simulink model "AttitudePlayground"  (R2024b)
settings: Solver=FixedStepAuto  StartTime=0.0  StopTime=inf  FixedStep=delta_t  RelTol=1e-3  EnableMultiTasking=on
values from neighbouring files (symbols this model uses):
  A = [eye(3), delta_t * eye(3) ... (first row only)    [AttitudePlayground_Vars.m]    (also in ParameterIdentification.m = [0 1)
  A_ESO = [1-l1_ESO, delta_t-l1_ESO*delta_t ... (first row only)    [AttitudePlayground_Vars.m]
  A_kalman = [1 delta_t ... (first row only)    [AttitudePlayground_Vars.m]    (also in ControlSystem_Vars.m)
  acc_sigma = 0.2 * calc_sigma(acc_pp)    [AttitudePlayground_Vars.m]    (also in ControlSystem_Vars.m)
  alpha_comp_pitch = calc_alpha(0.1, delta_t)    [AttitudePlayground_Vars.m]
  alpha_comp_roll = calc_alpha(0.1, delta_t)    [AttitudePlayground_Vars.m]
  alpha_comp_yaw = calc_alpha(1, delta_t)    [AttitudePlayground_Vars.m]
  B = zeros(6,3)    [AttitudePlayground_Vars.m]    (also in ParameterIdentification.m = [0)
  b_ESO = [b0_ESO*delta_t - l1_ESO*b0_ESO*delta_t ... (first row only)    [AttitudePlayground_Vars.m]
  bias_0 = [0, 0, 0]    [AttitudePlayground_Vars.m]
  bias_sigma = 0.000000001    (= 1e-09)    [AttitudePlayground_Vars.m]
  C = eye(6)    [AttitudePlayground_Vars.m]    (also in ParameterIdentification.m = [1 0])
  C_kalman = eye(2)    [AttitudePlayground_Vars.m]    (also in ControlSystem_Vars.m)
  delta_t = 0.01    [AttitudePlayground_Vars.m]    (also in ControlSystem_Vars.m; ParameterIdentification.m = t2 - t1)
  gyro_sigma = 1*((pi/180) * (0.07))    (= 0.0012217304764)    [AttitudePlayground_Vars.m]    (also in ControlSystem_Vars.m)
  gyro_sigma_3d = [1*gyro_sigma, 1*gyro_sigma, gyro_sigma]    [AttitudePlayground_Vars.m]    (also in ControlSystem_Vars.m)
  k_i_mahony = 0.0057    [AttitudePlayground_Vars.m]
  k_p_mahony = 0.42    [AttitudePlayground_Vars.m]
  l = [l1_ESO, l2_ESO]'    [AttitudePlayground_Vars.m]
  mag_sigma = 0.8 * calc_sigma(mag_pp)    [AttitudePlayground_Vars.m]
  P_0 = eye(4)    [AttitudePlayground_Vars.m]    (also in ControlSystem_Vars.m)
  P_0_gb = eye(7)    [AttitudePlayground_Vars.m]
  q_init = [cos(initial_yaw/2), 0, 0, sin(initial_yaw/2)]    [AttitudePlayground_Vars.m]
  q_sigma = 0.001    [AttitudePlayground_Vars.m]    (also in ControlSystem_Vars.m)
  R = 1.8 * diag([0.001396263^2, 0.0016580628^2, 0.05^2, ((pi/180) *              (0.05))^2, ((pi/180) * (0.07))^2, ((pi/180) * (0.07))^2])    [AttitudePlayground_Vars.m]    (also in ControlSystem_Vars.m = 0.015625)
  R_kalman = diag([(calc_sigma(0.8))^2, (0.07)^2])    [AttitudePlayground_Vars.m]    (also in ControlSystem_Vars.m)
  r_qekf = 1/sqrt(cos(magnetic_dip_angle_theta)^2 +      sin(magnetic_dip_angle_theta)^2)  * transpose([cos(magnetic_dip_angle_theta),0, sin(magnetic_dip_angle_theta)])    [AttitudePlayground_Vars.m]
  step_time = 10    [AttitudePlayground_Vars.m]
  tau_pitch_comp = 0.5    [AttitudePlayground_Vars.m]
  tau_roll_comp = 0.5    [AttitudePlayground_Vars.m]
  tau_yaw_comp = 3    [AttitudePlayground_Vars.m]
  Ts = delta_t    (= 0.01)    [AttitudePlayground_Vars.m]
  Ts2 = delta_t/2    (= 0.005)    [AttitudePlayground_Vars.m]
  Ts_IMU = delta_t    (= 0.01)    [AttitudePlayground_Vars.m]
  voltage_divider_Vout_max = 1.728    [AttitudePlayground_Vars.m]
undefined symbols (not defined in the file or in its folder): DiscIntNeverNeededParam, Discrete, Newton, Raphson, Time
libraries: simulink_extras x26, dspsigops x5, bbblueActuatorLib x4, ctrlSharedLib x2, matrix_library x2, dspmathops x2, dspstat3 x1, bbblueSensorLib x1, simulink x1, dspfdesign x1, bbblueBasicLib x1, vrlib x1
(part 2 of 3)

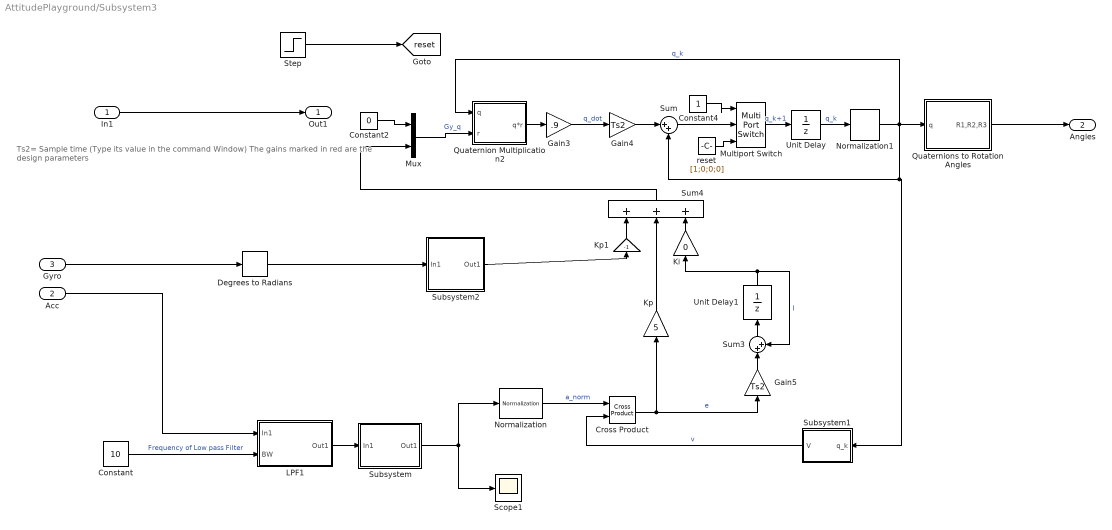
== system AttitudePlayground/Subsystem3 ==
  note: Ts2= Sample time (Type its value in the command Window)
      |
      | The gains marked in red are the design parameters
  In1 : Inport
  Acc : Inport  Port=2
  Gyro : Inport  Port=3
  Constant : Constant  Value=10
  Constant2 : Constant  Value=0
  Constant4 : Constant
  Cross Product : vrlib/Utilities/Cross Product
  Degrees to Radians : simulink_extras/Transformations/Degrees to Radians
  Gain3 : Gain  Gain=.9
  Gain4 : Gain  Gain=Ts2
  Gain5 : Gain  Gain=Ts2
  Ki : Gain  Gain=0
  Kp : Gain  Gain=5
  Kp1 : Gain  Gain=-1
  LPF1 : Subsystem
  Multiport Switch : MultiPortSwitch  Inputs=2  SaturateOnIntegerOverflow=off  InputSameDT=off
  Mux : Mux  Inputs=2
  Normalization : dspmathops/Normalization  NormType=Squared 2-norm  Bias=1e-10  NormOver=Each column  Dimension=1  roundingMode=Floor  overflowMode=off  accumDataTypeStr=Inherit: Same as product output  accumLastDataTypeStr=Inherit: Same as product output  outputDataTypeStr=Inherit: Same as product output  outputMin=[]  outputMax=[]  outputLastDataTypeStr=Inherit: Same as product output
  Normalization1 : dspmathops/Normalization  NormType=Squared 2-norm  Bias=1e-10  NormOver=Each column  Dimension=1  roundingMode=Floor  overflowMode=off  accumDataTypeStr=Inherit: Same as product output  accumLastDataTypeStr=Inherit: Same as product output  outputDataTypeStr=Inherit: Same as product output  outputMin=[]  outputMax=[]  outputLastDataTypeStr=Inherit: Same as product output
  Quaternion Multiplication2 : Subsystem
  Quaternions to Rotation Angles : Subsystem
  Scope1 : Scope
  Step : Step  Time=5  Before=2  SampleTime=delta_t
  Subsystem : Subsystem
  Subsystem1 : Subsystem
  Subsystem2 : Subsystem
  Sum : Sum  Inputs=|++
  Sum3 : Sum  Inputs=|++
  Sum4 : Sum  Inputs=+++
  Unit Delay : UnitDelay  InitialCondition=[1;0;0;0]  SampleTime=Ts  HasFrameUpgradeWarning=on
  Unit Delay1 : UnitDelay  InitialCondition=[0;0;0]  SampleTime=Ts  HasFrameUpgradeWarning=on
  reset : Constant  Value=[1;0;0;0]
  Out1 : Outport
  Angles : Outport  Port=2  VectorParamsAs1DForOutWhenUnconnected=off
  tag scope: reset=global
  wires:
  In1/1 -> Out1/1
  LPF1/1(Out1) -> Subsystem/1(In1)
  Sum4/1 -> Mux/2
  Gyro/1 -> Degrees to Radians/1
  Kp1/1 -> Sum4/1
  Ki/1 -> Sum4/3
  Unit Delay/1 -> Normalization1/1  "q_k"
  Subsystem2/1(Out1) -> Kp1/1
  reset/1 -> Multiport Switch/3
  Gain4/1 -> Sum/1
  Step/1 -> [reset]
  Unit Delay1/1 -> Ki/1, Sum3/2  "I"
  Constant4/1 -> Multiport Switch/1
  Sum/1 -> Multiport Switch/2
  Normalization/1 -> Cross Product/1  "a_norm"
  Constant/1 -> LPF1/2(BW)  "Frequency of Low pass Filter"
  Constant2/1 -> Mux/1
  Mux/1 -> Quaternion Multiplication2/2(r)  "Gy_q"
  Subsystem/1(Out1) -> Scope1/1, Normalization/1
  Gain3/1 -> Gain4/1  "q_dot"
  Quaternion Multiplication2/1(q*r) -> Gain3/1
  Degrees to Radians/1 -> Subsystem2/1(In1)
  Cross Product/1 -> Kp/1, Gain5/1  "e"
  Kp/1 -> Sum4/2
  Multiport Switch/1 -> Unit Delay/1  "q_k+1"
  Sum3/1 -> Unit Delay1/1
  Gain5/1 -> Sum3/1
  Subsystem1/1(V) -> Cross Product/2  "v"
  Acc/1 -> LPF1/1(In1)
  Quaternions to Rotation Angles/1(R1,R2,R3) -> Angles/1
  Normalization1/1 -> Quaternion Multiplication2/1(q), Quaternions to Rotation Angles/1(q), Subsystem1/1(q_k), Sum/2  "q_k"

== system AttitudePlayground/madgewick ==
  Gyroscope : Inport
  Out1 : Outport
  wires:
  Gyroscope/1 -> ?

== system AttitudePlayground/Angle_Accumulator_mat/Angle accumulator ==
  angle : Inport
  Bias : Bias  SaturateOnIntegerOverflow=off
  Constant4 : Constant
  Constant5 : Constant  Value=0
  Constant8 : Constant
  Constant9 : Constant  Value=0
  Gain : Gain  Gain=360
  Gain3 : Gain  Gain=-1
  Sum : Sum  Inputs=|++
  Sum1 : Sum  Inputs=|++
  Sum2 : Sum  Inputs=|-+
  Sum5 : Sum  Inputs=|++
  Sum6 : Sum  Inputs=+-|
  Switch : Switch  Criteria=u2 > Threshold  Threshold=180  SaturateOnIntegerOverflow=off  InputSameDT=off
  Switch1 : Switch  Criteria=u2 > Threshold  Threshold=180  SaturateOnIntegerOverflow=off  InputSameDT=off
  Unit Delay : UnitDelay  SampleTime=-1  HasFrameUpgradeWarning=on
  Unit Delay1 : UnitDelay  SampleTime=-1  HasFrameUpgradeWarning=on
  Unit Delay3 : UnitDelay  SampleTime=-1  HasFrameUpgradeWarning=on
  angle_acc : Outport
  wires:
  Sum1/1 -> Unit Delay/1, Sum6/1  "rot_amoun_fwt"
  Constant5/1 -> Switch/3
  Constant8/1 -> Switch1/1
  Sum5/1 -> Unit Delay3/1, Sum6/2
  Sum6/1 -> Gain/1
  Unit Delay/1 -> Sum1/2
  Constant4/1 -> Switch/1
  angle/1 -> Bias/1
  Unit Delay3/1 -> Sum5/2
  Switch/1 -> Sum1/1  "rot_done_fw"
  Sum2/1 -> Gain3/1, Switch/2
  Gain3/1 -> Switch1/2
  Unit Delay1/1 -> Sum2/2
  Sum/1 -> angle_acc/1  "abs_angle_deg"
  Switch1/1 -> Sum5/1  "rot_done_bw"
  Constant9/1 -> Switch1/3
  Gain/1 -> Sum/2
  Bias/1 -> Unit Delay1/1, Sum/1, Sum2/1

== system AttitudePlayground/Calculate RSME/Reset ==
  In1 : Inport  Partition=on  PartitionDimension=1  PartitionWidth=1  PartitionOffset=0
  For Each : ForEach  DisableCoverage=on
  Sample and Hold : dspsigops/Sample and Hold  trig=Rising edge  initCond=0  latchinput=off
  Step : Step  Time=step_time  SampleTime=0
  Sum : Sum  Inputs=|+-
  Out1 : Outport  ConcatenationDimension=1
  wires:
  In1/1 -> Sum/1, Sample and Hold/1
  Sample and Hold/1 -> Sum/2
  Step/1 -> Sample and Hold/Trigger
  Sum/1 -> Out1/1

== system AttitudePlayground/For Each Subsystem/Yaw accumulator ==
  yaw : Inport
  Bias : Bias  SaturateOnIntegerOverflow=off
  Constant4 : Constant
  Constant5 : Constant  Value=0
  Constant8 : Constant
  Constant9 : Constant  Value=0
  Gain : Gain  Gain=360
  Gain3 : Gain  Gain=-1
  Sum : Sum  Inputs=|++
  Sum1 : Sum  Inputs=|++
  Sum2 : Sum  Inputs=|-+
  Sum5 : Sum  Inputs=|++
  Sum6 : Sum  Inputs=+-|
  Switch : Switch  Criteria=u2 > Threshold  Threshold=180  SaturateOnIntegerOverflow=off  InputSameDT=off
  Switch1 : Switch  Criteria=u2 > Threshold  Threshold=180  SaturateOnIntegerOverflow=off  InputSameDT=off
  Unit Delay : UnitDelay  SampleTime=-1  HasFrameUpgradeWarning=on
  Unit Delay1 : UnitDelay  SampleTime=-1  HasFrameUpgradeWarning=on
  Unit Delay3 : UnitDelay  SampleTime=-1  HasFrameUpgradeWarning=on
  yaw_acc : Outport
  wires:
  Sum1/1 -> Unit Delay/1, Sum6/1  "rot_amoun_fwt"
  Constant5/1 -> Switch/3
  Constant8/1 -> Switch1/1
  Sum5/1 -> Unit Delay3/1, Sum6/2
  Sum6/1 -> Gain/1
  Unit Delay/1 -> Sum1/2
  Constant4/1 -> Switch/1
  yaw/1 -> Bias/1
  Unit Delay3/1 -> Sum5/2
  Switch/1 -> Sum1/1  "rot_done_fw"
  Sum2/1 -> Gain3/1, Switch/2
  Gain3/1 -> Switch1/2
  Unit Delay1/1 -> Sum2/2
  Sum/1 -> yaw_acc/1  "abs_angle_deg"
  Switch1/1 -> Sum5/1  "rot_done_bw"
  Constant9/1 -> Switch1/3
  Gain/1 -> Sum/2
  Bias/1 -> Unit Delay1/1, Sum/1, Sum2/1

== system AttitudePlayground/For Each Subsystem2/Yaw accumulator ==
  yaw : Inport
  Bias : Bias  SaturateOnIntegerOverflow=off
  Constant4 : Constant
  Constant5 : Constant  Value=0
  Constant8 : Constant
  Constant9 : Constant  Value=0
  Gain : Gain  Gain=360
  Gain3 : Gain  Gain=-1
  Sum : Sum  Inputs=|++
  Sum1 : Sum  Inputs=|++
  Sum2 : Sum  Inputs=|-+
  Sum5 : Sum  Inputs=|++
  Sum6 : Sum  Inputs=+-|
  Switch : Switch  Criteria=u2 > Threshold  Threshold=180  SaturateOnIntegerOverflow=off  InputSameDT=off
  Switch1 : Switch  Criteria=u2 > Threshold  Threshold=180  SaturateOnIntegerOverflow=off  InputSameDT=off
  Unit Delay : UnitDelay  SampleTime=-1  HasFrameUpgradeWarning=on
  Unit Delay1 : UnitDelay  SampleTime=-1  HasFrameUpgradeWarning=on
  Unit Delay3 : UnitDelay  SampleTime=-1  HasFrameUpgradeWarning=on
  yaw_acc : Outport
  wires:
  Sum1/1 -> Unit Delay/1, Sum6/1  "rot_amoun_fwt"
  Constant5/1 -> Switch/3
  Constant8/1 -> Switch1/1
  Sum5/1 -> Unit Delay3/1, Sum6/2
  Sum6/1 -> Gain/1
  Unit Delay/1 -> Sum1/2
  Constant4/1 -> Switch/1
  yaw/1 -> Bias/1
  Unit Delay3/1 -> Sum5/2
  Switch/1 -> Sum1/1  "rot_done_fw"
  Sum2/1 -> Gain3/1, Switch/2
  Gain3/1 -> Switch1/2
  Unit Delay1/1 -> Sum2/2
  Sum/1 -> yaw_acc/1  "abs_angle_deg"
  Switch1/1 -> Sum5/1  "rot_done_bw"
  Constant9/1 -> Switch1/3
  Gain/1 -> Sum/2
  Bias/1 -> Unit Delay1/1, Sum/1, Sum2/1

== system AttitudePlayground/Leightweight-Kalman/Yaw accumulator1 ==
  yaw : Inport
  Bias : Bias  SaturateOnIntegerOverflow=off
  Constant4 : Constant
  Constant5 : Constant  Value=0
  Constant8 : Constant
  Constant9 : Constant  Value=0
  Gain : Gain  Gain=360
  Gain3 : Gain  Gain=-1
  Sum : Sum  Inputs=|++
  Sum1 : Sum  Inputs=|++
  Sum2 : Sum  Inputs=|-+
  Sum5 : Sum  Inputs=|++
  Sum6 : Sum  Inputs=+-|
  Switch : Switch  Criteria=u2 > Threshold  Threshold=180  SaturateOnIntegerOverflow=off  InputSameDT=off
  Switch1 : Switch  Criteria=u2 > Threshold  Threshold=180  SaturateOnIntegerOverflow=off  InputSameDT=off
  Unit Delay : UnitDelay  SampleTime=-1  HasFrameUpgradeWarning=on
  Unit Delay1 : UnitDelay  SampleTime=-1  HasFrameUpgradeWarning=on
  Unit Delay3 : UnitDelay  SampleTime=-1  HasFrameUpgradeWarning=on
  yaw_acc : Outport
  wires:
  Sum1/1 -> Unit Delay/1, Sum6/1  "rot_amoun_fwt"
  Constant5/1 -> Switch/3
  Constant8/1 -> Switch1/1
  Sum5/1 -> Unit Delay3/1, Sum6/2
  Sum6/1 -> Gain/1
  Unit Delay/1 -> Sum1/2
  Constant4/1 -> Switch/1
  yaw/1 -> Bias/1
  Unit Delay3/1 -> Sum5/2
  Switch/1 -> Sum1/1  "rot_done_fw"
  Sum2/1 -> Gain3/1, Switch/2
  Gain3/1 -> Switch1/2
  Unit Delay1/1 -> Sum2/2
  Sum/1 -> yaw_acc/1  "abs_angle_deg"
  Switch1/1 -> Sum5/1  "rot_done_bw"
  Constant9/1 -> Switch1/3
  Gain/1 -> Sum/2
  Bias/1 -> Unit Delay1/1, Sum/1, Sum2/1

== system AttitudePlayground/Mahony Backup/Gyro - Bias - Removal ==
  In1 : Inport
  Constant1 : Constant  Value=0
  Constant3 : Constant
  Constant5 : Constant  Value=0
  Multiport Switch1 : MultiPortSwitch  Inputs=2  SaturateOnIntegerOverflow=off  InputSameDT=off
  Multiport Switch2 : MultiPortSwitch  Inputs=2  SaturateOnIntegerOverflow=off  InputSameDT=off
  Step : Step  Time=5  Before=2  SampleTime=Ts_IMU
  Subsystem3 : Subsystem
  Sum1 : Sum  Inputs=|+-
  Out1 : Outport  VectorParamsAs1DForOutWhenUnconnected=off
  tag scope: reset=global
  wires:
  [reset] -> Multiport Switch2/1
  In1/1 -> Subsystem3/1(Gyro), Sum1/1
  Constant3/1 -> Multiport Switch1/3
  Constant1/1 -> Multiport Switch1/2
  Sum1/1 -> Multiport Switch2/2
  Constant5/1 -> Multiport Switch2/3
  Multiport Switch1/1 -> Subsystem3/2(Switch)
  Subsystem3/1(Bias) -> Sum1/2
  [reset] -> Multiport Switch1/1
  Multiport Switch2/1 -> Out1/1
  Step/1 -> [reset]

== system AttitudePlayground/Mahony+Bias-Estimator/BIAS-ESO ==
  u : Inport
  Yaw_Fused : Inport  Port=2
  Gain : Gain  Gain=l
  Gain1 : Gain  Gain=b_ESO
  Gain2 : Gain  Gain=A_ESO  Multiplication=Matrix(K*u)
  Sum : Sum  Inputs=|++
  Sum1 : Sum  Inputs=++|
  Unit Delay : UnitDelay  SampleTime=delta_t  HasFrameUpgradeWarning=on
  Bias : Outport
  wires:
  Yaw_Fused/1 -> Gain/1
  u/1 -> Gain1/1
  Gain1/1 -> Sum/1
  Gain2/1 -> Sum/2
  Sum/1 -> Unit Delay/1
  Unit Delay/1 -> Sum1/1
  Gain/1 -> Sum1/2
  Sum1/1 -> Bias/1, Gain2/1  "x_hat"

== system AttitudePlayground/Mahony+Bias-Estimator/Gyro - Bias - Removal ==
  In1 : Inport
  Constant1 : Constant  Value=0
  Constant3 : Constant
  Constant5 : Constant  Value=0
  Multiport Switch1 : MultiPortSwitch  Inputs=2  SaturateOnIntegerOverflow=off  InputSameDT=off
  Multiport Switch2 : MultiPortSwitch  Inputs=2  SaturateOnIntegerOverflow=off  InputSameDT=off
  Step : Step  Time=step_time  Before=2  SampleTime=Ts_IMU
  Subsystem3 : Subsystem
  Sum1 : Sum  Inputs=|+-
  Out1 : Outport  VectorParamsAs1DForOutWhenUnconnected=off
  wires:
  Step/1 -> Multiport Switch2/1, Multiport Switch1/1
  In1/1 -> Subsystem3/1(Gyro), Sum1/1
  Constant3/1 -> Multiport Switch1/3
  Constant1/1 -> Multiport Switch1/2
  Sum1/1 -> Multiport Switch2/2
  Constant5/1 -> Multiport Switch2/3
  Multiport Switch1/1 -> Subsystem3/2(Switch)
  Subsystem3/1(Bias) -> Sum1/2
  Multiport Switch2/1 -> Out1/1

== system AttitudePlayground/Subsystem3/LPF1 ==
  In1 : Inport
  BW : Inport  Port=2
  Demux1 : Demux  Outputs=3
  LPF : Subsystem
  LPF1 : Subsystem
  LPF2 : Subsystem
  Mux1 : Mux  Inputs=3
  Out1 : Outport  VectorParamsAs1DForOutWhenUnconnected=off
  wires:
  In1/1 -> Demux1/1
  Demux1/2 -> LPF1/1(In)
  LPF1/1(Out1) -> Mux1/2
  BW/1 -> LPF2/2(BW), LPF1/2(BW), LPF/2(BW)
  LPF2/1(Out1) -> Mux1/3
  Demux1/3 -> LPF2/1(In)
  LPF/1(Out1) -> Mux1/1
  Mux1/1 -> Out1/1
  Demux1/1 -> LPF/1(In)

== system AttitudePlayground/Subsystem3/Quaternion Multiplication2 ==
  q : Inport  Unit=1
  r : Inport  Port=2  Unit=1
  Fcn : Fcn  Expr=u(5)*u(1) - u(6)*u(2) - u(7)*u(3) - u(8)*u(4)
  Fcn1 : Fcn  Expr=u(5)*u(2) + u(6)*u(1) - u(7)*u(4) + u(8)*u(3)
  Fcn2 : Fcn  Expr=u(5)*u(3) + u(6)*u(4) + u(7)*u(1) - u(8)*u(2)
  Fcn3 : Fcn  Expr=u(5)*u(4) - u(6)*u(3) + u(7)*u(2) + u(8)*u(1)
  Mux1 : Mux  Inputs=2
  Mux2 : Mux
  q*r : Outport  Unit=1  VectorParamsAs1DForOutWhenUnconnected=off
  wires:
  Mux1/1 -> Fcn3/1, Fcn2/1, Fcn/1, Fcn1/1
  Fcn/1 -> Mux2/1  "t0"
  Fcn1/1 -> Mux2/2  "t1"
  Fcn2/1 -> Mux2/3  "t2"
  Fcn3/1 -> Mux2/4  "t3"
  q/1 -> Mux1/1
  r/1 -> Mux1/2
  Mux2/1 -> q*r/1

== system AttitudePlayground/Subsystem3/Quaternions to Rotation Angles ==
  q : Inport  Unit=1
  Angle Calculation : Subsystem
  Quaternion Normalize : Subsystem
  fcn1 : Fcn  Expr=2*(u[2]*u[3] + u[1]*u[4])
  fcn2 : Fcn  Expr=u[1]*u[1] + u[2]*u[2] - u[3]*u[3] - u[4]*u[4]
  fcn3 : Fcn  Expr=-2*(u[2]*u[4] - u[1]*u[3])
  fcn4 : Fcn  Expr=2*(u[3]*u[4] + u[1]*u[2])
  fcn5 : Fcn  Expr=u[1]*u[1] - u[2]*u[2] - u[3]*u[3] + u[4]*u[4]
  R1,R2,R3 : Outport  Unit=rad  VectorParamsAs1DForOutWhenUnconnected=off
  wires:
  Quaternion Normalize/1(normal(q)) -> fcn3/1, fcn4/1, fcn5/1, fcn2/1, fcn1/1
  q/1 -> Angle Calculation/1(q), Quaternion Normalize/1(q)
  fcn2/1 -> Angle Calculation/3(r12)
  fcn3/1 -> Angle Calculation/4(r21)
  fcn5/1 -> Angle Calculation/6(r32)
  fcn4/1 -> Angle Calculation/5(In4)
  Angle Calculation/1(R1,R2,R3) -> R1,R2,R3/1
  fcn1/1 -> Angle Calculation/2(r11)

== system AttitudePlayground/Subsystem3/Subsystem ==
  In1 : Inport
  Constant6 : Constant  Value=0
  Constant7 : Constant
  Multiport Switch3 : MultiPortSwitch  Inputs=2  SaturateOnIntegerOverflow=off  InputSameDT=off
  Subsystem3 : Subsystem
  Sum2 : Sum  Inputs=|+-
  Out1 : Outport  VectorParamsAs1DForOutWhenUnconnected=off
  wires:
  Sum2/1 -> Out1/1
  Constant6/1 -> Multiport Switch3/2
  Subsystem3/1(Bias) -> Sum2/2
  In1/1 -> Sum2/1, Subsystem3/1(Accel)
  Multiport Switch3/1 -> Subsystem3/2(Switch)
  Constant7/1 -> Multiport Switch3/3
  [reset] -> Multiport Switch3/1

== system AttitudePlayground/Subsystem3/Subsystem1 ==
  q_k : Inport
  Fcn : Fcn  Expr=2*(u(2)*u(4)-u(1)*u(3))
  Fcn1 : Fcn  Expr=2*(u(1)*u(2)+u(3)*u(4))
  Fcn2 : Fcn  Expr=2*(0.5-u(2)^2-u(3)^2)
  Mux1 : Mux  Inputs=3
  V : Outport  VectorParamsAs1DForOutWhenUnconnected=off
  wires:
  Mux1/1 -> V/1
  Fcn2/1 -> Mux1/3
  Fcn1/1 -> Mux1/2
  q_k/1 -> Fcn2/1, Fcn1/1, Fcn/1
  Fcn/1 -> Mux1/1

== system AttitudePlayground/Subsystem3/Subsystem2 ==
  In1 : Inport
  Constant1 : Constant  Value=0
  Constant3 : Constant
  Constant5 : Constant  Value=0
  Multiport Switch1 : MultiPortSwitch  Inputs=2  SaturateOnIntegerOverflow=off  InputSameDT=off
  Multiport Switch2 : MultiPortSwitch  Inputs=2  SaturateOnIntegerOverflow=off  InputSameDT=off
  Subsystem3 : Subsystem
  Sum1 : Sum  Inputs=|+-
  Out1 : Outport  VectorParamsAs1DForOutWhenUnconnected=off
  wires:
  [reset] -> Multiport Switch2/1
  In1/1 -> Subsystem3/1(Gyro), Sum1/1
  Constant3/1 -> Multiport Switch1/3
  Constant1/1 -> Multiport Switch1/2
  Sum1/1 -> Multiport Switch2/2
  Constant5/1 -> Multiport Switch2/3
  Multiport Switch1/1 -> Subsystem3/2(Switch)
  Subsystem3/1(Bias) -> Sum1/2
  [reset] -> Multiport Switch1/1
  Multiport Switch2/1 -> Out1/1

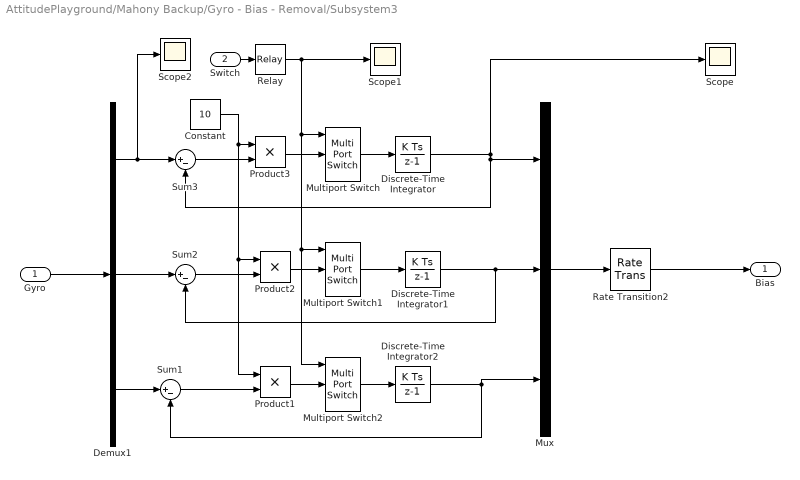
== system AttitudePlayground/Mahony Backup/Gyro - Bias - Removal/Subsystem3 ==
  Gyro : Inport
  Switch : Inport  Port=2
  Constant : Constant  Value=10
  Demux1 : Demux  Outputs=3
  Discrete-Time Integrator : DiscreteIntegrator  SampleTime=Ts_IMU  ICPrevOutput=DiscIntNeverNeededParam  ICPrevScaledInput=DiscIntNeverNeededParam
  Discrete-Time Integrator1 : DiscreteIntegrator  SampleTime=Ts_IMU  ICPrevOutput=DiscIntNeverNeededParam  ICPrevScaledInput=DiscIntNeverNeededParam
  Discrete-Time Integrator2 : DiscreteIntegrator  SampleTime=Ts_IMU  ICPrevOutput=DiscIntNeverNeededParam  ICPrevScaledInput=DiscIntNeverNeededParam
  Multiport Switch : MultiPortSwitch  Inputs=2  SaturateOnIntegerOverflow=off  InputSameDT=off
  Multiport Switch1 : MultiPortSwitch  Inputs=2  SaturateOnIntegerOverflow=off  InputSameDT=off
  Multiport Switch2 : MultiPortSwitch  Inputs=2  SaturateOnIntegerOverflow=off  InputSameDT=off
  Mux : Mux  Inputs=3
  Product1 : Product
  Product2 : Product
  Product3 : Product
  Rate Transition2 : RateTransition  OutPortSampleTime=Ts_IMU
  Relay : Relay  OnSwitchValue=.5  OffSwitchValue=.5  OffOutputValue=2
  Scope : Scope
  Scope1 : Scope
  Scope2 : Scope
  Sum1 : Sum  Inputs=|+-
  Sum2 : Sum  Inputs=|+-
  Sum3 : Sum  Inputs=|+-
  Bias : Outport  VectorParamsAs1DForOutWhenUnconnected=off
  wires:
  Gyro/1 -> Demux1/1
  Demux1/3 -> Sum1/1
  Product1/1 -> Multiport Switch2/2
  Sum1/1 -> Product1/2
  Multiport Switch2/1 -> Discrete-Time Integrator2/1
  Multiport Switch1/1 -> Discrete-Time Integrator1/1
  Sum2/1 -> Product2/2
  Product2/1 -> Multiport Switch1/2
  Demux1/2 -> Sum2/1
  Demux1/1 -> Scope2/1, Sum3/1
  Product3/1 -> Multiport Switch/2
  Sum3/1 -> Product3/2
  Discrete-Time Integrator/1 -> Sum3/2, Mux/1, Scope/1
  Constant/1 -> Product3/1, Product2/1, Product1/1
  Mux/1 -> Rate Transition2/1
  Multiport Switch/1 -> Discrete-Time Integrator/1
  Switch/1 -> Relay/1
  Relay/1 -> Scope1/1, Multiport Switch1/1, Multiport Switch2/1, Multiport Switch/1
  Rate Transition2/1 -> Bias/1
  Discrete-Time Integrator1/1 -> Sum2/2, Mux/2
  Discrete-Time Integrator2/1 -> Sum1/2, Mux/3

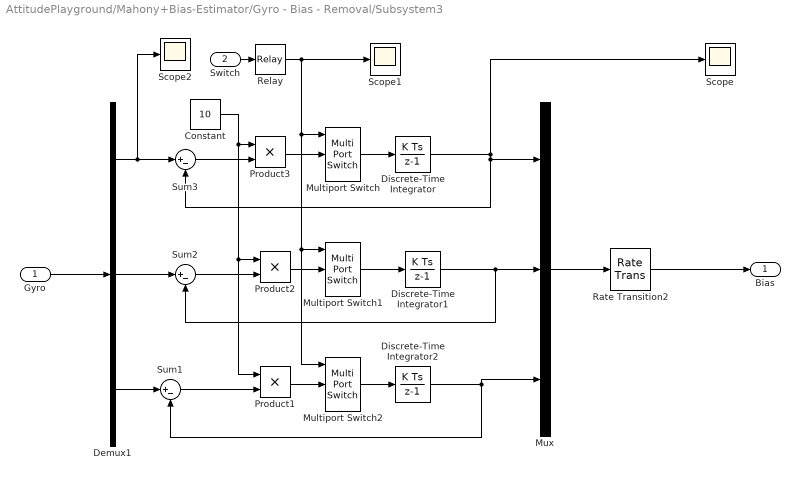
== system AttitudePlayground/Mahony+Bias-Estimator/Gyro - Bias - Removal/Subsystem3 ==
  Gyro : Inport
  Switch : Inport  Port=2
  Constant : Constant  Value=10
  Demux1 : Demux  Outputs=3
  Discrete-Time Integrator : DiscreteIntegrator  SampleTime=Ts_IMU  ICPrevOutput=DiscIntNeverNeededParam  ICPrevScaledInput=DiscIntNeverNeededParam
  Discrete-Time Integrator1 : DiscreteIntegrator  SampleTime=Ts_IMU  ICPrevOutput=DiscIntNeverNeededParam  ICPrevScaledInput=DiscIntNeverNeededParam
  Discrete-Time Integrator2 : DiscreteIntegrator  SampleTime=Ts_IMU  ICPrevOutput=DiscIntNeverNeededParam  ICPrevScaledInput=DiscIntNeverNeededParam
  Multiport Switch : MultiPortSwitch  Inputs=2  SaturateOnIntegerOverflow=off  InputSameDT=off
  Multiport Switch1 : MultiPortSwitch  Inputs=2  SaturateOnIntegerOverflow=off  InputSameDT=off
  Multiport Switch2 : MultiPortSwitch  Inputs=2  SaturateOnIntegerOverflow=off  InputSameDT=off
  Mux : Mux  Inputs=3
  Product1 : Product
  Product2 : Product
  Product3 : Product
  Rate Transition2 : RateTransition  OutPortSampleTime=Ts_IMU
  Relay : Relay  OnSwitchValue=.5  OffSwitchValue=.5  OffOutputValue=2
  Scope : Scope
  Scope1 : Scope
  Scope2 : Scope
  Sum1 : Sum  Inputs=|+-
  Sum2 : Sum  Inputs=|+-
  Sum3 : Sum  Inputs=|+-
  Bias : Outport  VectorParamsAs1DForOutWhenUnconnected=off
  wires:
  Gyro/1 -> Demux1/1
  Demux1/3 -> Sum1/1
  Product1/1 -> Multiport Switch2/2
  Sum1/1 -> Product1/2
  Multiport Switch2/1 -> Discrete-Time Integrator2/1
  Multiport Switch1/1 -> Discrete-Time Integrator1/1
  Sum2/1 -> Product2/2
  Product2/1 -> Multiport Switch1/2
  Demux1/2 -> Sum2/1
  Demux1/1 -> Scope2/1, Sum3/1
  Product3/1 -> Multiport Switch/2
  Sum3/1 -> Product3/2
  Discrete-Time Integrator/1 -> Sum3/2, Mux/1, Scope/1
  Constant/1 -> Product3/1, Product2/1, Product1/1
  Mux/1 -> Rate Transition2/1
  Multiport Switch/1 -> Discrete-Time Integrator/1
  Switch/1 -> Relay/1
  Relay/1 -> Scope1/1, Multiport Switch1/1, Multiport Switch2/1, Multiport Switch/1
  Rate Transition2/1 -> Bias/1
  Discrete-Time Integrator1/1 -> Sum2/2, Mux/2
  Discrete-Time Integrator2/1 -> Sum1/2, Mux/3

== system AttitudePlayground/Subsystem3/LPF1/LPF ==
  In : Inport
  BW : Inport  Port=2
  Discrete-Time Integrator : DiscreteIntegrator  SampleTime=Ts  ICPrevOutput=DiscIntNeverNeededParam  ICPrevScaledInput=DiscIntNeverNeededParam
  Product : Product
  Sum2 : Sum  Inputs=|+-
  Out1 : Outport  VectorParamsAs1DForOutWhenUnconnected=off
  wires:
  In/1 -> Sum2/1
  Sum2/1 -> Product/2
  Discrete-Time Integrator/1 -> Out1/1, Sum2/2
  Product/1 -> Discrete-Time Integrator/1
  BW/1 -> Product/1

== system AttitudePlayground/Subsystem3/LPF1/LPF1 ==
  In : Inport
  BW : Inport  Port=2
  Discrete-Time Integrator : DiscreteIntegrator  SampleTime=Ts  ICPrevOutput=DiscIntNeverNeededParam  ICPrevScaledInput=DiscIntNeverNeededParam
  Product : Product
  Sum2 : Sum  Inputs=|+-
  Out1 : Outport  VectorParamsAs1DForOutWhenUnconnected=off
  wires:
  BW/1 -> Product/1
  Product/1 -> Discrete-Time Integrator/1
  Discrete-Time Integrator/1 -> Sum2/2, Out1/1
  Sum2/1 -> Product/2
  In/1 -> Sum2/1

== system AttitudePlayground/Subsystem3/LPF1/LPF2 ==
  In : Inport
  BW : Inport  Port=2
  Discrete-Time Integrator : DiscreteIntegrator  SampleTime=Ts  ICPrevOutput=DiscIntNeverNeededParam  ICPrevScaledInput=DiscIntNeverNeededParam
  Product : Product
  Sum2 : Sum  Inputs=|+-
  Out1 : Outport  VectorParamsAs1DForOutWhenUnconnected=off
  wires:
  In/1 -> Sum2/1
  Sum2/1 -> Product/2
  Discrete-Time Integrator/1 -> Out1/1, Sum2/2
  Product/1 -> Discrete-Time Integrator/1
  BW/1 -> Product/1

== system AttitudePlayground/Subsystem3/Quaternions to Rotation Angles/Angle Calculation ==
  q : Inport
  r11 : Inport  Port=2
  r12 : Inport  Port=3
  r21 : Inport  Port=4
  In4 : Inport  Port=5
  r32 : Inport  Port=6
  Terminator : Terminator
  Trigonometric Function1 : Trigonometry  Operator=atan2
  Trigonometric Function3 : Trigonometry  Operator=atan2
  Vector Concatenate : Concatenate  NumInputs=3
  trigFcn : Trigonometry  Operator=asin
  R1,R2,R3 : Outport  VectorParamsAs1DForOutWhenUnconnected=off
  wires:
  Vector Concatenate/1 -> R1,R2,R3/1
  r11/1 -> Trigonometric Function1/1
  In4/1 -> Trigonometric Function3/1
  trigFcn/1 -> Vector Concatenate/2  "r2"
  r32/1 -> Trigonometric Function3/2
  r21/1 -> trigFcn/1
  Trigonometric Function3/1 -> Vector Concatenate/3  "r3"
  q/1 -> Terminator/1
  Trigonometric Function1/1 -> Vector Concatenate/1  "r1"
  r12/1 -> Trigonometric Function1/2

== system AttitudePlayground/Subsystem3/Quaternions to Rotation Angles/Quaternion Normalize ==
  q : Inport  Unit=1
  Demux : Demux
  Mux : Mux
  Product{,1..3} (4 alike) : Product  Inputs=*/
  Quaternion Modulus : Subsystem
  normal(q) : Outport  Unit=1  VectorParamsAs1DForOutWhenUnconnected=off
  wires:
  Product/1 -> Mux/1
  Product1/1 -> Mux/2
  Demux/1 -> Product/1
  Demux/2 -> Product1/1
  q/1 -> Quaternion Modulus/1(q), Demux/1
  Demux/4 -> Product3/1
  Mux/1 -> normal(q)/1
  Demux/3 -> Product2/1
  Product3/1 -> Mux/4
  Product2/1 -> Mux/3
  Quaternion Modulus/1(|q|) -> Product3/2, Product2/2, Product/2, Product1/2

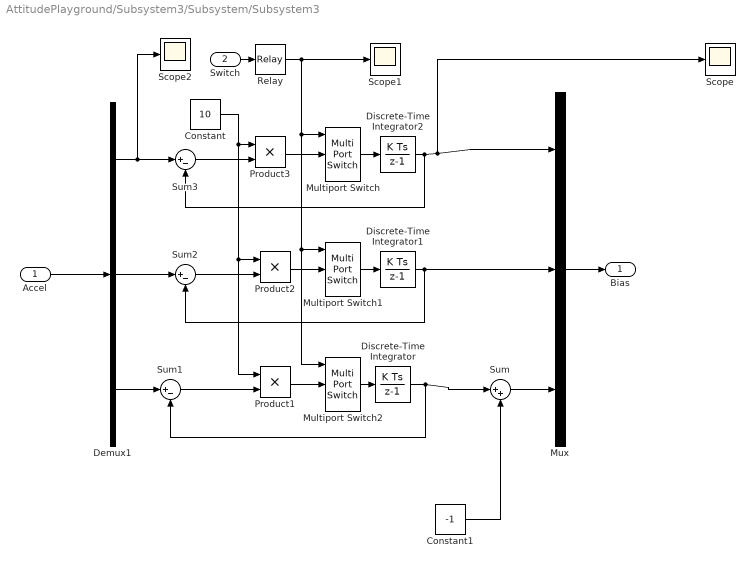
== system AttitudePlayground/Subsystem3/Subsystem/Subsystem3 ==
  Accel : Inport
  Switch : Inport  Port=2
  Constant : Constant  Value=10
  Constant1 : Constant  Value=-1
  Demux1 : Demux  Outputs=3
  Discrete-Time Integrator : DiscreteIntegrator  SampleTime=delta_t  ICPrevOutput=DiscIntNeverNeededParam  ICPrevScaledInput=DiscIntNeverNeededParam
  Discrete-Time Integrator1 : DiscreteIntegrator  SampleTime=delta_t  ICPrevOutput=DiscIntNeverNeededParam  ICPrevScaledInput=DiscIntNeverNeededParam
  Discrete-Time Integrator2 : DiscreteIntegrator  SampleTime=delta_t  ICPrevOutput=DiscIntNeverNeededParam  ICPrevScaledInput=DiscIntNeverNeededParam
  Multiport Switch : MultiPortSwitch  Inputs=2  SaturateOnIntegerOverflow=off  InputSameDT=off
  Multiport Switch1 : MultiPortSwitch  Inputs=2  SaturateOnIntegerOverflow=off  InputSameDT=off
  Multiport Switch2 : MultiPortSwitch  Inputs=2  SaturateOnIntegerOverflow=off  InputSameDT=off
  Mux : Mux  Inputs=3
  Product1 : Product
  Product2 : Product
  Product3 : Product
  Relay : Relay  OnSwitchValue=.5  OffSwitchValue=.5  OffOutputValue=2
  Scope : Scope
  Scope1 : Scope
  Scope2 : Scope
  Sum : Sum  Inputs=|++
  Sum1 : Sum  Inputs=|+-
  Sum2 : Sum  Inputs=|+-
  Sum3 : Sum  Inputs=|+-
  Bias : Outport  VectorParamsAs1DForOutWhenUnconnected=off
  wires:
  Accel/1 -> Demux1/1
  Demux1/3 -> Sum1/1
  Product1/1 -> Multiport Switch2/2
  Sum1/1 -> Product1/2
  Discrete-Time Integrator/1 -> Sum/1, Sum1/2
  Discrete-Time Integrator1/1 -> Mux/2, Sum2/2
  Sum2/1 -> Product2/2
  Product2/1 -> Multiport Switch1/2
  Demux1/2 -> Sum2/1
  Demux1/1 -> Scope2/1, Sum3/1
  Product3/1 -> Multiport Switch/2
  Sum3/1 -> Product3/2
  Discrete-Time Integrator2/1 -> Scope/1, Mux/1, Sum3/2
  Constant/1 -> Product3/1, Product2/1, Product1/1
  Mux/1 -> Bias/1
  Multiport Switch/1 -> Discrete-Time Integrator2/1
  Multiport Switch1/1 -> Discrete-Time Integrator1/1
  Multiport Switch2/1 -> Discrete-Time Integrator/1
  Switch/1 -> Relay/1
  Relay/1 -> Scope1/1, Multiport Switch1/1, Multiport Switch2/1, Multiport Switch/1
  Sum/1 -> Mux/3
  Constant1/1 -> Sum/2

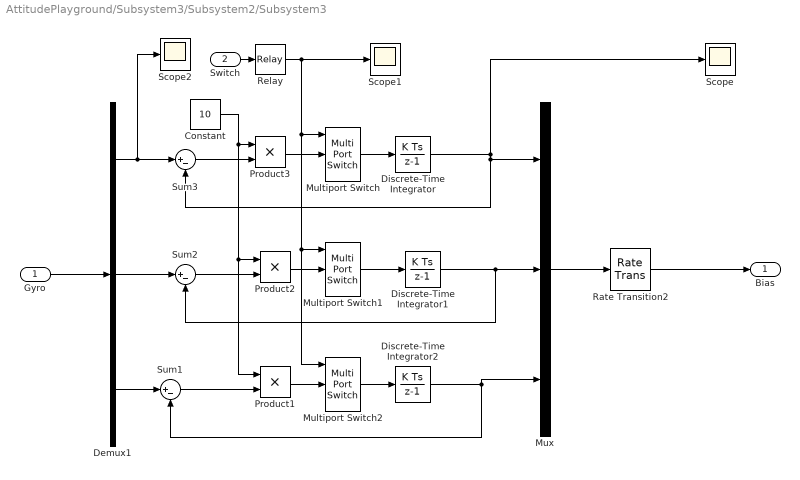
== system AttitudePlayground/Subsystem3/Subsystem2/Subsystem3 ==
  Gyro : Inport
  Switch : Inport  Port=2
  Constant : Constant  Value=10
  Demux1 : Demux  Outputs=3
  Discrete-Time Integrator : DiscreteIntegrator  SampleTime=delta_t  ICPrevOutput=DiscIntNeverNeededParam  ICPrevScaledInput=DiscIntNeverNeededParam
  Discrete-Time Integrator1 : DiscreteIntegrator  SampleTime=delta_t  ICPrevOutput=DiscIntNeverNeededParam  ICPrevScaledInput=DiscIntNeverNeededParam
  Discrete-Time Integrator2 : DiscreteIntegrator  SampleTime=delta_t  ICPrevOutput=DiscIntNeverNeededParam  ICPrevScaledInput=DiscIntNeverNeededParam
  Multiport Switch : MultiPortSwitch  Inputs=2  SaturateOnIntegerOverflow=off  InputSameDT=off
  Multiport Switch1 : MultiPortSwitch  Inputs=2  SaturateOnIntegerOverflow=off  InputSameDT=off
  Multiport Switch2 : MultiPortSwitch  Inputs=2  SaturateOnIntegerOverflow=off  InputSameDT=off
  Mux : Mux  Inputs=3
  Product1 : Product
  Product2 : Product
  Product3 : Product
  Rate Transition2 : RateTransition  OutPortSampleTime=delta_t
  Relay : Relay  OnSwitchValue=.5  OffSwitchValue=.5  OffOutputValue=2
  Scope : Scope
  Scope1 : Scope
  Scope2 : Scope
  Sum1 : Sum  Inputs=|+-
  Sum2 : Sum  Inputs=|+-
  Sum3 : Sum  Inputs=|+-
  Bias : Outport  VectorParamsAs1DForOutWhenUnconnected=off
  wires:
  Gyro/1 -> Demux1/1
  Demux1/3 -> Sum1/1
  Product1/1 -> Multiport Switch2/2
  Sum1/1 -> Product1/2
  Multiport Switch2/1 -> Discrete-Time Integrator2/1
  Multiport Switch1/1 -> Discrete-Time Integrator1/1
  Sum2/1 -> Product2/2
  Product2/1 -> Multiport Switch1/2
  Demux1/2 -> Sum2/1
  Demux1/1 -> Scope2/1, Sum3/1
  Product3/1 -> Multiport Switch/2
  Sum3/1 -> Product3/2
  Discrete-Time Integrator/1 -> Sum3/2, Mux/1, Scope/1
  Constant/1 -> Product3/1, Product2/1, Product1/1
  Mux/1 -> Rate Transition2/1
  Multiport Switch/1 -> Discrete-Time Integrator/1
  Switch/1 -> Relay/1
  Relay/1 -> Scope1/1, Multiport Switch1/1, Multiport Switch2/1, Multiport Switch/1
  Rate Transition2/1 -> Bias/1
  Discrete-Time Integrator1/1 -> Sum2/2, Mux/2
  Discrete-Time Integrator2/1 -> Sum1/2, Mux/3

== system AttitudePlayground/Subsystem3/Quaternions to Rotation Angles/Quaternion Normalize/Quaternion Modulus ==
  q : Inport  Unit=1
  Quaternion Norm : Subsystem
  sqrt : Sqrt  AlgorithmType=Newton-Raphson
  |q| : Outport  Unit=1  VectorParamsAs1DForOutWhenUnconnected=off
  wires:
  sqrt/1 -> |q|/1
  Quaternion Norm/1(norm(q)) -> sqrt/1
  q/1 -> Quaternion Norm/1(q)

== system AttitudePlayground/Subsystem3/Quaternions to Rotation Angles/Quaternion Normalize/Quaternion Modulus/Quaternion Norm ==
  q : Inport  Unit=1
  Demux : Demux
  Product{,1..3} (4 alike) : Product
  Sum : Sum  Inputs=4
  norm(q) : Outport  Unit=1  VectorParamsAs1DForOutWhenUnconnected=off
  wires:
  Demux/3 -> Product2/1, Product2/2
  q/1 -> Demux/1
  Sum/1 -> norm(q)/1
  Demux/2 -> Product1/1, Product1/2
  Product/1 -> Sum/1
  Product2/1 -> Sum/3
  Product3/1 -> Sum/4
  Demux/4 -> Product3/1, Product3/2
  Demux/1 -> Product/1, Product/2
  Product1/1 -> Sum/2

== matlab function AttitudePlayground/Mahony Backup/MATLAB Function1 ==
  data: euler output; omega input; delta_t input; quat_mem input; quaternion_tplus output
function [euler, quaternion_tplus] = fcn(omega, delta_t, quat_mem)

q0 = quat_mem(1);
q1 = quat_mem(2);
q2 = quat_mem(3);
q3 = quat_mem(4);

omega_x = omega(1);
omega_y = omega(2);
omega_z = omega(3);

q0_tp = q0 + delta_t/2 * (-omega_x * q1 - omega_y * q2 - omega_z * q3);
q1_tp = q1 + delta_t/2 * ( omega_x * q0 + omega_z * q2 - omega_y * q3);
q2_tp = q2 + delta_t/2 * ( omega_y * q0 - omega_z * q1 + omega_z * q3);
q3_tp = q3 + delta_t/2 * ( omega_z * q0 + omega_y * q1 - omega_x * q2);

quaternion_tplus = [q0_tp, q1_tp, q2_tp, q3_tp];

roll = atan((2 * (q0_tp*q1_tp + q2_tp*q3_tp))/(1 - 2*(q1_tp^2 + q2_tp^2)));
pitch = asin(2 * (q0_tp*q2_tp - q1_tp*q3_tp));
yaw = atan2((2 * (q0_tp*q3_tp + q1_tp*q2_tp)),(1 - 2*(q2_tp^2 + q3_tp^2)));

euler = [roll, pitch, yaw];

== matlab function AttitudePlayground/Mahony Backup/MATLAB Function2 ==
  data: q input; v_b output
function v_b = fcn(q)

q0 = q(1);
q1 = q(2);
q2 = q(3);
q3 = q(4);
v_b = [2*(q1*q3 - q0*q2);
       2*(q0*q1 + q2*q3);
       1 - 2*(q1^2 + q2^2)];

== matlab function AttitudePlayground/Mahony Backup/convert to quat ==
  data: u input; y output
function y = fcn(u)

y = eul2quat([u(1) u(2) u(3)]);

== matlab function AttitudePlayground/Mahony Backup/normalize quat ==
  data: q input; y output
function y = fcn(q)
q0 = q(1);
q1 = q(2);
q2 = q(3);
q3 = q(4);
y = quatnormalize([q0 q1 q2 q3]);

== matlab function AttitudePlayground/Mahony Backup/normalize_g_b ==
  data: g_b input; g_b_norm output
function g_b_norm = fcn(g_b)

g_b_norm = g_b / norm(g_b);

== matlab function AttitudePlayground/Quarternion EKF/normalize_g_b ==
  data: v input; v_norm output
function v_norm = normalize_vec(v)

v_norm = v / norm(v);

== matlab function AttitudePlayground/Quarternion EKF/normalize_vec ==
  data: v input; v_norm output
function v_norm = normalize_vec(v)

v_norm = v / norm(v);

== matlab function AttitudePlayground/Quarternion EKF/MATLAB Function ==
  data: quat_in input; euler output
function euler = to_euler(quat_in)

q0 = quat_in(1);
q1 = quat_in(2);
q2 = quat_in(3);
q3 = quat_in(4);

roll = atan((2 * (q0*q1 + q2*q3))/(1 - 2*(q1^2 + q2^2)));
pitch = asin(2 * (q0*q2 - q1*q3));
yaw = atan2((2 * (q0*q3 + q1*q2)),(1 - 2*(q2^2 + q3^2)));

euler = [roll; pitch; yaw];

== matlab function AttitudePlayground/Quarternion with Gyro Bias Estimation & Mag/MATLAB Function ==
  data: quat_in input; euler output
function euler = to_euler(quat_in)

q0 = quat_in(1);
q1 = quat_in(2);
q2 = quat_in(3);
q3 = quat_in(4);

roll = atan((2 * (q0*q1 + q2*q3))/(1 - 2*(q1^2 + q2^2)));
pitch = asin(2 * (q0*q2 - q1*q3));
yaw = atan2((2 * (q0*q3 + q1*q2)),(1 - 2*(q2^2 + q3^2)));

euler = [roll; pitch; yaw];

== matlab function AttitudePlayground/Quarternion with Gyro Bias Estimation & Mag/Predict ==
  data: omega input; state_in input; x_t_dash output; delta_t input; P_t_dash output; P_t_ input; gyro_sigma input; bias_sigma input
function [x_t_dash, P_t_dash] = Predict(omega, state_in, delta_t, P_t_, gyro_sigma, bias_sigma)

q0 = state_in(1);
q1 = state_in(2);
q2 = state_in(3);
q3 = state_in(4);
bx = state_in(5);
by = state_in(6);
bz = state_in(7);

omega_x = omega(1);
omega_y = omega(2);
omega_z = omega(3);

x = [q0; q1; q2; q3; bx; by; bz];

dt2 = delta_t/2;
F = [1  -dt2*(omega_x-bx) -dt2*(omega_y-by) -dt2*(omega_z-bz)     dt2*q1  dt2*q2  dt2*q3;
    dt2*(omega_x-bx)    1  dt2*(omega_z-bz) -dt2*(omega_y-by)    -dt2*q0  dt2*q3 -dt2*q2;
    dt2*(omega_y-by)   -dt2*(omega_z-bz)   1 dt2*(omega_x-bx)    -dt2*q3 -dt2*q0  dt2*q1;
    dt2*(omega_z-bz)    dt2*(omega_y-by) -dt2*(omega_x-bx)  1     dt2*q2 -dt2*q1 -dt2*q0;
                            zeros(3,4)                                    eye(3)       ;];

x_t_dash = F*x;
q_t_dash = quatnormalize([x_t_dash(1), x_t_dash(2), x_t_dash(3), x_t_dash(4)]);
x_t_dash = [q_t_dash(1), q_t_dash(2), q_t_dash(3), q_t_dash(4), x_t_dash(5), x_t_dash(6), x_t_dash(7)]';

W = dt2 * [-q1 -q2 -q3;
            q0 -q3  q2;
            q3  q0 -q1;
            -q2 q1  q0;
             zeros(3,3)]; 

Q = gyro_sigma^2 * eye(3);
Q_bias = [zeros(4,7);
          zeros(3,4) bias_sigma^2*eye(3)];

Q_t =  W*Q*W' + Q_bias;

P_t_dash = F * P_t_ * F' + Q_t;


%{
q0_out = q0 + delta_t/2 * (-omega_x * q1 - omega_y * q2 - omega_z * q3);
q1_out = q1 + delta_t/2 * ( omega_x * q0 + omega_z * q2 - omega_y * q3);
q2_out = q2 + delta_t/2 * ( omega_y * q0 - omega_z * q1 + omega_z * q3);
q3_out = q3 + delta_t/2 * ( omega_z * q0 + omega_y * q1 - omega_x * q2);
%}

== matlab function AttitudePlayground/Quarternion with Gyro Bias Estimation & Mag/Update ==
  data: accel input; mag input; q_t output; b_t output; state_in input; r input; acc_sigma input; mag_sigma input; P_t output; P_t_dash input
function [q_t, b_t, P_t]   = Update(accel, mag, state_in, r, acc_sigma, mag_sigma, P_t_dash)

q0 = state_in(1);
q1 = state_in(2);
q2 = state_in(3);
q3 = state_in(4);
bx = state_in(5);
by = state_in(6);
bz = state_in(7);

x_t_dash = [q0; q1; q2; q3; bx; by; bz];

z_t = [accel(1);
       accel(2);
       accel(3);
         mag(1);
         mag(2);
         mag(3);];

rx = r(1);
ry = r(2);
rz = r(3);
gx = 0;
gy = 0;
gz = 1;

R = [acc_sigma^2 * eye(3) zeros(3);
    zeros(3)     mag_sigma^2 * eye(3)];


h = 2 * [
    gx * (1/2 - q2^2 - q3^2) + gy * (q0*q3 + q1*q2) + gz * (q1*q3 - q0*q2);
    gx * (q1*q2 - q0*q3) + gy * (1/2 - q1^2 - q3^2) + gz * (q0*q1 + q2*q3);
    gx * (q0*q2 + q1*q3) + gy * (q2*q3 - q0*q1) + gz * (1/2 - q1^2 - q2^2);
    rx * (1/2 - q2^2 - q3^2) + ry * (q0*q3 + q1*q2) + rz * (q1*q3 - q0*q2);
    rx * (q1*q2 - q0*q3) + ry * (1/2 - q1^2 - q3^2) + rz * (q0*q1 + q2*q3);
    rx * (q0*q2 + q1*q3) + ry * (q2*q3 - q0*q1) + rz * (1/2 - q1^2 - q2^2)
];

H = 2 * [
    gx*q0 + gy*q3 - gz*q2,  gx*q1 + gy*q2 + gz*q3, -gx*q2 + gy*q1 - gz*q0, -gx*q3 + gy*q0 + gz*q1, 0, 0, 0;
   -gx*q3 + gy*q0 + gz*q1,  gx*q2 - gy*q1 + gz*q0,  gx*q1 + gy*q2 + gz*q3, -gx*q0 - gy*q3 + gz*q2, 0, 0, 0;
    gx*q2 - gy*q1 + gz*q0,  gx*q3 - gy*q0 - gz*q1,  gx*q0 + gy*q3 - gz*q2,  gx*q1 + gy*q2 + gz*q3, 0, 0, 0;
    rx*q0 + ry*q3 - rz*q2,  rx*q1 + ry*q2 + rz*q3, -rx*q2 + ry*q1 - rz*q0, -rx*q3 + ry*q0 + rz*q1, 0, 0, 0;
   -rx*q3 + ry*q0 + rz*q1,  rx*q2 - ry*q1 + rz*q0,  rx*q1 + ry*q2 + rz*q3, -rx*q0 - ry*q3 + rz*q2, 0, 0, 0;
    rx*q2 - ry*q1 + rz*q0,  rx*q3 - ry*q0 - rz*q1,  rx*q0 + ry*q3 - rz*q2,  rx*q1 + ry*q2 + rz*q3, 0, 0, 0
];

v_t = z_t - h;

S_t = H * P_t_dash * H' + R;
K_t = P_t_dash * H' * S_t^-1;

x_t = x_t_dash + K_t*v_t;

q_t = quatnormalize(transpose(x_t(1:4)));
b_t = transpose(x_t(5:7));

P_t = (eye(7) - K_t*H) * P_t_dash;

== matlab function AttitudePlayground/Quarternion with Gyro Bias Estimation & Mag/normalize_g_b ==
  data: v input; v_norm output
function v_norm = normalize_vec(v)

v_norm = v / norm(v);

== matlab function AttitudePlayground/Quarternion with Gyro Bias Estimation & Mag/normalize_vec ==
  data: v input; v_norm output
function v_norm = normalize_vec(v)

v_norm = v / norm(v);

== matlab function AttitudePlayground/Quarternion with Gyro Bias Estimation & no Mag/MATLAB Function ==
  data: quat_in input; euler output
function euler = to_euler(quat_in)

q0 = quat_in(1);
q1 = quat_in(2);
q2 = quat_in(3);
q3 = quat_in(4);

roll = atan((2 * (q0*q1 + q2*q3))/(1 - 2*(q1^2 + q2^2)));
pitch = asin(2 * (q0*q2 - q1*q3));
yaw = atan2((2 * (q0*q3 + q1*q2)),(1 - 2*(q2^2 + q3^2)));

euler = [roll; pitch; yaw];

== matlab function AttitudePlayground/Quarternion with Gyro Bias Estimation & no Mag/Predict ==
  data: state_in input; x_t_dash output; omega input; delta_t input; P_t_dash output; P_t_ input; gyro_sigma input; bias_sigma input
function [x_t_dash, P_t_dash] = Predict(state_in, omega, delta_t, P_t_, gyro_sigma, bias_sigma)

q0 = state_in(1);
q1 = state_in(2);
q2 = state_in(3);
q3 = state_in(4);
bx = state_in(5);
by = state_in(6);
bz = state_in(7);

omega_x = omega(1);
omega_y = omega(2);
omega_z = omega(3);

x = [q0; q1; q2; q3; bx; by; bz];

dt2 = delta_t/2;
F = [1  -dt2*(omega_x-bx) -dt2*(omega_y-by) -dt2*(omega_z-bz)     dt2*q1  dt2*q2  dt2*q3;
    dt2*(omega_x-bx)    1  dt2*(omega_z-bz) -dt2*(omega_y-by)    -dt2*q0  dt2*q3 -dt2*q2;
    dt2*(omega_y-by)   -dt2*(omega_z-bz)   1 dt2*(omega_x-bx)    -dt2*q3 -dt2*q0  dt2*q1;
    dt2*(omega_z-bz)    dt2*(omega_y-by) -dt2*(omega_x-bx)  1     dt2*q2 -dt2*q1 -dt2*q0;
                            zeros(3,4)                                    eye(3)       ;];

x_t_dash = F*x;

W = dt2 * [-q1 -q2 -q3;
            q0 -q3  q2;
            q3  q0 -q1;
            -q2 q1  q0;
             zeros(3,3)]; 

Q = gyro_sigma^2 * eye(3);
Q_bias = [zeros(4,7);
          zeros(3,4) bias_sigma^2*eye(3)];

Q_t =  W*Q*W' + Q_bias;

P_t_dash = F * P_t_ * F' + Q_t;


%{
q0_out = q0 + delta_t/2 * (-omega_x * q1 - omega_y * q2 - omega_z * q3);
q1_out = q1 + delta_t/2 * ( omega_x * q0 + omega_z * q2 - omega_y * q3);
q2_out = q2 + delta_t/2 * ( omega_y * q0 - omega_z * q1 + omega_z * q3);
q3_out = q3 + delta_t/2 * ( omega_z * q0 + omega_y * q1 - omega_x * q2);
%}

== matlab function AttitudePlayground/Angles from Accel + Mag/MATLAB Function1 ==
  data: a_x input; a_y input; pitch output; a_z input; roll input
function pitch = calc_pitch(a_x, a_y, a_z, roll)

pitch = atan(-a_x / (a_y * sin(roll) + a_z * cos(roll)));

== matlab function AttitudePlayground/Quarternion with Gyro Bias Estimation & no Mag/Update ==
  data: accel input; q_t output; b_t output; state_in input; acc_sigma input; P_t output; P_t_dash input
function [q_t, b_t, P_t]   = Update(accel, state_in, acc_sigma, P_t_dash)

q0 = state_in(1);
q1 = state_in(2);
q2 = state_in(3);
q3 = state_in(4);
bx = state_in(5);
by = state_in(6);
bz = state_in(7);

x_t_dash = [q0; q1; q2; q3; bx; by; bz];

z_t = [accel(1);
       accel(2);
       accel(3)];

gx = 0;
gy = 0;
gz = 1;

R = acc_sigma^2 * eye(3);


h = 2 * [
    gx * (1/2 - q2^2 - q3^2) + gy * (q0*q3 + q1*q2) + gz * (q1*q3 - q0*q2);
    gx * (q1*q2 - q0*q3) + gy * (1/2 - q1^2 - q3^2) + gz * (q0*q1 + q2*q3);
    gx * (q0*q2 + q1*q3) + gy * (q2*q3 - q0*q1) + gz * (1/2 - q1^2 - q2^2);
];

H = 2 * [
    gx*q0 + gy*q3 - gz*q2,  gx*q1 + gy*q2 + gz*q3, -gx*q2 + gy*q1 - gz*q0, -gx*q3 + gy*q0 + gz*q1, 0, 0, 0;
   -gx*q3 + gy*q0 + gz*q1,  gx*q2 - gy*q1 + gz*q0,  gx*q1 + gy*q2 + gz*q3, -gx*q0 - gy*q3 + gz*q2, 0, 0, 0;
    gx*q2 - gy*q1 + gz*q0,  gx*q3 - gy*q0 - gz*q1,  gx*q0 + gy*q3 - gz*q2,  gx*q1 + gy*q2 + gz*q3, 0, 0, 0;
];

v_t = z_t - h;

S_t = H * P_t_dash * H' + R;
K_t = P_t_dash * H' * inv(S_t);

x_t = x_t_dash + K_t*v_t;

q_t = quatnormalize(transpose(x_t(1:4)));
b_t = transpose(x_t(5:7));

P_t = (eye(7) - K_t*H) * P_t_dash;

== matlab function AttitudePlayground/Quarternion with Gyro Bias Estimation & no Mag/normalize_g_b ==
  data: v input; v_norm output
function v_norm = normalize_vec(v)

v_norm = v / norm(v);

== matlab function AttitudePlayground/MATLAB Function ==
  data: yaw_init_rad input; q_init output
function q_init = calc_q_init(yaw_init_rad)

q_init = [cos(yaw_init_rad/2), 0, 0, sin(yaw_init_rad/2)];

== matlab function AttitudePlayground/MATLAB Function1 ==
  data: quat_in input; euler output
function euler = to_euler(quat_in)

q0 = quat_in(1);
q1 = quat_in(2);
q2 = quat_in(3);
q3 = quat_in(4);

roll = atan((2 * (q0*q1 + q2*q3))/(1 - 2*(q1^2 + q2^2)));
pitch = asin(2 * (q0*q2 - q1*q3));
yaw = atan2((2 * (q0*q3 + q1*q2)),(1 - 2*(q2^2 + q3^2)));

euler = [roll; pitch; yaw];

== matlab function AttitudePlayground/Mahony+Bias-Estimator/MATLAB Function ==
  data: yaw_est input; omega_yaw_est output; prev_yaw_est input; delta_t input
function omega_yaw_est = est_omega_yaw(yaw_est,prev_yaw_est,delta_t)

omega_yaw_est = (yaw_est - prev_yaw_est) / delta_t;

== matlab function AttitudePlayground/Quarternion EKF + Amfitrack/MATLAB Function ==
  data: quat_in input; euler output
function euler = to_euler(quat_in)

q0 = quat_in(1);
q1 = quat_in(2);
q2 = quat_in(3);
q3 = quat_in(4);

roll = atan((2 * (q0*q1 + q2*q3))/(1 - 2*(q1^2 + q2^2)));
pitch = asin(2 * (q0*q2 - q1*q3));
yaw = atan2((2 * (q0*q3 + q1*q2)),(1 - 2*(q2^2 + q3^2)));

euler = [roll; pitch; yaw];

== matlab function AttitudePlayground/Quarternion EKF + Amfitrack/Predict ==
  data: quat_in input; q_t_dash output; omega input; delta_t input; P_t_dash output; P_t_ input; gyro_sigma input
function [q_t_dash, P_t_dash] = Predict(quat_in, omega, delta_t, P_t_, gyro_sigma)

q0 = quat_in(1);
q1 = quat_in(2);
q2 = quat_in(3);
q3 = quat_in(4);

omega_x = omega(1);
omega_y = omega(2);
omega_z = omega(3);

R_gyro = [gyro_sigma(1)^2 0 0;
          0 gyro_sigma(2)^2 0;
          0 0 gyro_sigma(3)^2;];

q0_out = q0 + delta_t/2 * (-omega_x * q1 - omega_y * q2 - omega_z * q3);
q1_out = q1 + delta_t/2 * ( omega_x * q0 - omega_y * q3 + omega_z * q2);
q2_out = q2 + delta_t/2 * ( omega_x * q3 + omega_y * q0 - omega_z * q1);
q3_out = q3 + delta_t/2 * (-omega_x * q2 + omega_y * q1 + omega_z * q0);

q_t_dash = quatnormalize([q0_out, q1_out, q2_out, q3_out]);

dt2 = delta_t/2;

F = [1  -dt2*omega_x -dt2*omega_y -dt2*omega_z;
    dt2*omega_x    1  dt2*omega_z  dt2*omega_y;
    dt2*omega_y   -dt2*omega_z   1 dt2*omega_x;
    dt2*omega_z    dt2*omega_y -dt2*omega_x  1;
    ];


W = dt2 * [-q1 -q2 -q3;
            q0 -q3  q2;
            q3  q0 -q1;
            -q2 q1  q0]; 

Q_t =  W* R_gyro * W';

P_t_dash = F * P_t_ * F' + Q_t;

== matlab function AttitudePlayground/Quarternion EKF + Amfitrack/Update ==
  data: accel input; q_meas input; q_t output; quat_in input; acc_sigma input; q_sigma input; P_t output; P_t_dash input
function [q_t, P_t]   = Update(accel, q_meas, quat_in, acc_sigma, q_sigma, P_t_dash)

q0 = quat_in(1);
q1 = quat_in(2);
q2 = quat_in(3);
q3 = quat_in(4);

q_t_dash = [q0; q1; q2; q3];

z_t = [accel(1);
       accel(2);
       accel(3);
         q_meas(1);
         q_meas(2);
         q_meas(3);
         q_meas(4)];

gx = 0;
gy = 0;
gz = 1;

R = [acc_sigma^2 * eye(3) zeros(3,4);
    zeros(4,3)     q_sigma^2 * eye(4)];


h = [
    2*(gx * (1/2 - q2^2 - q3^2) + gy * (q0*q3 + q1*q2) + gz * (q1*q3 - q0*q2));
    2*(gx * (q1*q2 - q0*q3) + gy * (1/2 - q1^2 - q3^2) + gz * (q0*q1 + q2*q3));
    2*(gx * (q0*q2 + q1*q3) + gy * (q2*q3 - q0*q1) + gz * (1/2 - q1^2 - q2^2));
                                    q0                                     ;
                                    q1                                     ;
                                    q2                                     ;
                                    q3                                     ;
];

H = 2 * [
    gx*q0 + gy*q3 - gz*q2,  gx*q1 + gy*q2 + gz*q3, -gx*q2 + gy*q1 - gz*q0, -gx*q3 + gy*q0 + gz*q1;
   -gx*q3 + gy*q0 + gz*q1,  gx*q2 - gy*q1 + gz*q0,  gx*q1 + gy*q2 + gz*q3, -gx*q0 - gy*q3 + gz*q2;
    gx*q2 - gy*q1 + gz*q0,  gx*q3 - gy*q0 - gz*q1,  gx*q0 + gy*q3 - gz*q2,  gx*q1 + gy*q2 + gz*q3;
                                            
                                                0.5*eye(4)
];

v_t = z_t - h;

S_t = H * P_t_dash * transpose(H) + R;
K_t = P_t_dash * transpose(H) * inv(S_t);

q_t = quatnormalize(transpose(q_t_dash + K_t*v_t));

P_t = (eye(4) - K_t*H) * P_t_dash;

== matlab function AttitudePlayground/Quarternion EKF + Amfitrack/normalize_g_b ==
  data: v input; v_norm output
function v_norm = normalize_vec(v)

v_norm = v / norm(v);

== matlab function AttitudePlayground/Quarternion EKF + Amfitrack (Yaw Only)/MATLAB Function ==
  data: quat_in input; euler output
function euler = to_euler(quat_in)

q0 = quat_in(1);
q1 = quat_in(2);
q2 = quat_in(3);
q3 = quat_in(4);

roll = atan((2 * (q0*q1 + q2*q3))/(1 - 2*(q1^2 + q2^2)));
pitch = asin(2 * (q0*q2 - q1*q3));
yaw = atan2((2 * (q0*q3 + q1*q2)),(1 - 2*(q2^2 + q3^2)));

euler = [roll; pitch; yaw];

== matlab function AttitudePlayground/Quarternion EKF + Amfitrack (Yaw Only)/Predict ==
  data: quat_in input; q_t_dash output; omega input; delta_t input; P_t_dash output; P_t_ input; gyro_sigma input
function [q_t_dash, P_t_dash] = Predict(quat_in, omega, delta_t, P_t_, gyro_sigma)

q0 = quat_in(1);
q1 = quat_in(2);
q2 = quat_in(3);
q3 = quat_in(4);

omega_x = omega(1);
omega_y = omega(2);
omega_z = omega(3);

R_gyro = [gyro_sigma(1)^2 0 0;
          0 gyro_sigma(2)^2 0;
          0 0 gyro_sigma(3)^2;];

q0_out = q0 + delta_t/2 * (-omega_x * q1 - omega_y * q2 - omega_z * q3);
q1_out = q1 + delta_t/2 * ( omega_x * q0 - omega_y * q3 + omega_z * q2);
q2_out = q2 + delta_t/2 * ( omega_x * q3 + omega_y * q0 - omega_z * q1);
q3_out = q3 + delta_t/2 * (-omega_x * q2 + omega_y * q1 + omega_z * q0);

q_t_dash = quatnormalize([q0_out, q1_out, q2_out, q3_out]);

dt2 = delta_t/2;

F = [1  -dt2*omega_x -dt2*omega_y -dt2*omega_z;
    dt2*omega_x    1  dt2*omega_z  dt2*omega_y;
    dt2*omega_y   -dt2*omega_z   1 dt2*omega_x;
    dt2*omega_z    dt2*omega_y -dt2*omega_x  1;
    ];


W = dt2 * [-q1 -q2 -q3;
            q0 -q3  q2;
            q3  q0 -q1;
            -q2 q1  q0]; 

Q_t =  W* R_gyro * W';

P_t_dash = F * P_t_ * F' + Q_t;

== matlab function AttitudePlayground/Angles from Accel + Mag/MATLAB Function ==
  data: a_y input; roll output; a_z input
function roll = calc_roll(a_y, a_z)

roll = atan(a_y / a_z);
